simulink model "DynamicSystemFinal"  (R2021a)
settings: Solver=VariableStepAuto  StartTime=0.0  StopTime=300  RelTol=1e-3
values from neighbouring files (symbols this model uses):
  res = zeros(1, 2)    [AutonomousVehicle.m]    (also in trajectory_final_2.m)
  speed = zeros(K-1,1)    [AutonomousVehicle.m]    (also in trajectory_final_2.m)
undefined symbols (not defined in the file or in its folder): DiscIntNeverNeededParam
libraries: simulink x5, pid_lib x2, dspswit3 x1, mcbcontrolslib x1
settings Model: Creator=admin  LastModifiedBy=admin

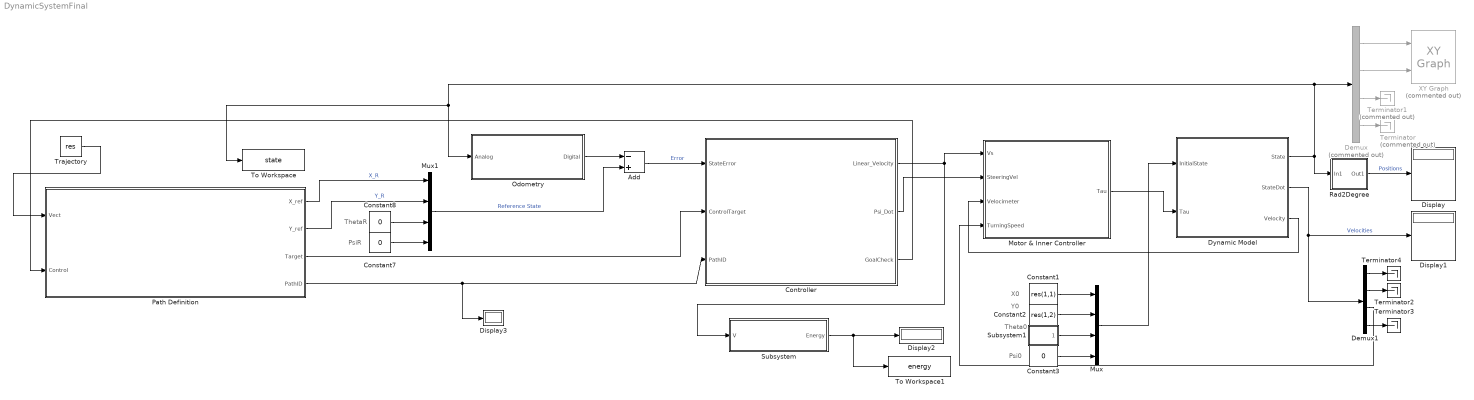
== system DynamicSystemFinal ==
  note: PsiR
  note: ThetaR
  note: Psi0
  note: Theta0
  note: X0
  note: Y0
  Add : Sum  Inputs=-+
  Constant1 : Constant  Value=res(1,1)  VectorParams1D=off  SampleTime=0.001
  Constant2 : Constant  Value=res(1,2)  SampleTime=0.001
  Constant3 : Constant  Value=0  SampleTime=0.001
  Constant7 : Constant  Value=0  SampleTime=0.001
  Constant8 : Constant  Value=0  SampleTime=0.001
  Controller : Subsystem
  Demux : Demux  Commented=on
  Demux1 : Demux
  Display{,1..3} (4 alike) : Display
  Dynamic Model : Subsystem
  Motor & Inner Controller : Subsystem
  Mux : Mux
  Mux1 : Mux
  Odometry : Subsystem
  Path Definition : Subsystem
  Rad2Degree : Subsystem
  Subsystem : Subsystem
  Subsystem1 : Subsystem
  Terminator : Terminator  Commented=on
  Terminator1 : Terminator  Commented=on
  Terminator2 : Terminator
  Terminator3 : Terminator
  Terminator4 : Terminator
  To Workspace : ToWorkspace  VariableName=state  SampleTime=0.001
      settings: Save2DSignal=2-D array (concatenate along first dimension)
  To Workspace1 : ToWorkspace  VariableName=energy  SaveFormat=Timeseries  SampleTime=0.001
      settings: MaxDataPoints=1
  Trajectory : Constant  Value=res
  XY Graph : simulink/Sinks/XY Graph  Commented=on  xmin=0  xmax=400  ymin=0  ymax=700  st=inf
  wires:
  Path Definition/4(PathID) -> Controller/3(PathID), Display3/1
  Demux/3 -> Terminator1/1
  Path Definition/3(Target) -> Controller/2(ControlTarget)
  Path Definition/1(X_ref) -> Mux1/1  "X_R"
  Add/1 -> Controller/1(StateError)  "Error"
  Controller/2(Psi_Dot) -> Motor & Inner Controller/2(SteeringVel)
  Dynamic Model/1(State) -> Rad2Degree/1(In1), Odometry/1(Analog), To Workspace/1, Demux/1
  Controller/1(Linear_Velocity) -> Motor & Inner Controller/1(Vs), Subsystem/1(V)
  Odometry/1(Digital) -> Add/1
  Constant2/1 -> Mux/2
  Rad2Degree/1(Out1) -> Display/1  "Positions"
  Mux1/1 -> Add/2  "Reference State"
  Path Definition/2(Y_ref) -> Mux1/2  "Y_R"
  Demux/4 -> Terminator/1
  Trajectory/1 -> Path Definition/1(Vect)
  Demux/1 -> XY Graph/1
  Subsystem/1(Energy) -> To Workspace1/1, Display2/1
  Demux/2 -> XY Graph/2
  Constant8/1 -> Mux1/3
  Mux/1 -> Dynamic Model/1(InitialState)
  Subsystem1/1(Theta0) -> Mux/3
  Constant7/1 -> Mux1/4
  Controller/3(GoalCheck) -> Path Definition/2(Control)
  Constant1/1 -> Mux/1
  Dynamic Model/2(StateDot) -> Demux1/1, Display1/1  "Velocities"
  Constant3/1 -> Mux/4
  Motor & Inner Controller/1(Tau) -> Dynamic Model/2(Tau)
  Dynamic Model/3(Velocity) -> Motor & Inner Controller/3(Velocimeter)
  Demux1/4 -> Terminator3/1
  Demux1/2 -> Terminator2/1
  Demux1/1 -> Terminator4/1
  Demux1/3 -> Motor & Inner Controller/4(TurningSpeed)

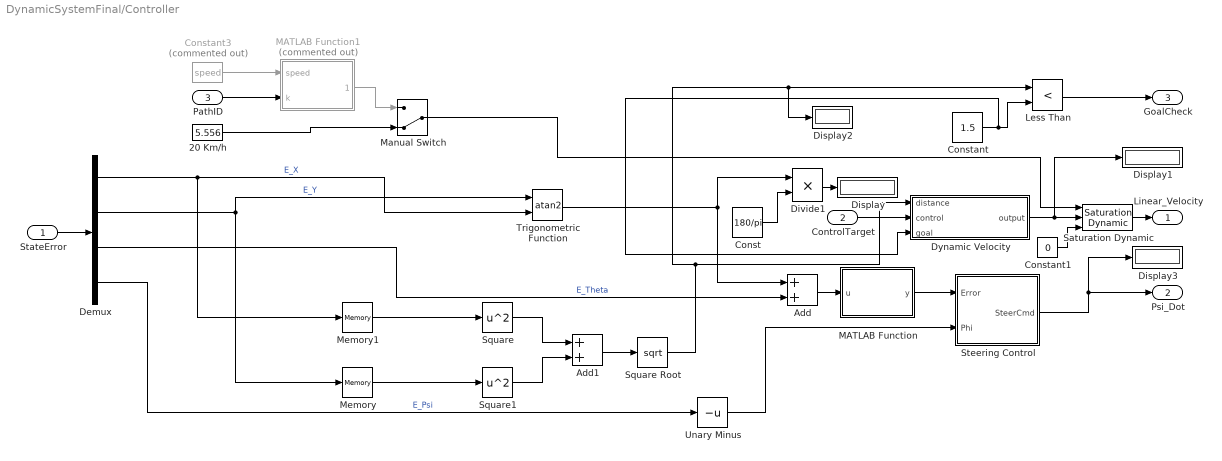
== system DynamicSystemFinal/Controller ==
  StateError : Inport
  ControlTarget : Inport  Port=2
  PathID : Inport  Port=3
  20 Km/h : Constant  Value=5.556
  Add : Sum
  Add1 : Sum
  Const : Constant  Value=180/pi
  Constant : Constant  Value=1.5  SampleTime=0.001
  Constant1 : Constant  Value=0
  Constant3 : Constant  Commented=on  Value=speed
  Demux : Demux
  Display{,1..3} (4 alike) : Display
  Divide1 : Product  Inputs=**
  Dynamic Velocity : Subsystem
  Less Than : RelationalOperator  Operator=<  OutDataTypeStr=boolean  RndMeth=Simplest
  MATLAB Function : MATLAB Function  TreatAsAtomicUnit=on
  MATLAB Function1 : MATLAB Function  Commented=on  TreatAsAtomicUnit=on
  Manual Switch : ManualSwitch  CurrentSetting=0
  Memory : Memory
  Memory1 : Memory
  Saturation Dynamic : simulink/Discontinuities/Saturation Dynamic  OutMin=[]  OutMax=[]  OutDataTypeStr=Inherit: Same as second input  OutDataType=fixdt(1, 16)  OutScaling=2^-10  DoSatur=off
  Square : Math  Operator=square  SaturateOnIntegerOverflow=on
  Square Root : Sqrt  SaturateOnIntegerOverflow=on
  Square1 : Math  Operator=square  SaturateOnIntegerOverflow=on
  Steering Control : Subsystem
  Trigonometric Function : Trigonometry  Operator=atan2
  Unary Minus : UnaryMinus
  Linear_Velocity : Outport
  Psi_Dot : Outport  Port=2
  GoalCheck : Outport  Port=3
  wires:
  StateError/1 -> Demux/1
  Demux/2 -> Trigonometric Function/1, Memory/1  "E_Y"
  Demux/3 -> Add/2  "E_Theta"
  Demux/1 -> Trigonometric Function/2, Memory1/1  "E_X"
  Constant/1 -> Dynamic Velocity/3(goal), Less Than/2
  Less Than/1 -> GoalCheck/1
  Square/1 -> Add1/1
  Square1/1 -> Add1/2
  Add1/1 -> Square Root/1
  Add/1 -> MATLAB Function/1(u)
  Const/1 -> Divide1/2
  Divide1/1 -> Display/1
  Square Root/1 -> Dynamic Velocity/1(distance), Less Than/1, Display2/1
  Dynamic Velocity/1(output) -> Display1/1, Saturation Dynamic/2
  ControlTarget/1 -> Dynamic Velocity/2(control)
  Memory/1 -> Square1/1
  Memory1/1 -> Square/1
  Saturation Dynamic/1 -> Linear_Velocity/1
  Constant1/1 -> Saturation Dynamic/3
  Manual Switch/1 -> Saturation Dynamic/1
  20 Km/h/1 -> Manual Switch/2
  Constant3/1 -> MATLAB Function1/1(speed)
  PathID/1 -> MATLAB Function1/2(k)
  MATLAB Function1/1(max_vel) -> Manual Switch/1
  Trigonometric Function/1 -> Divide1/1, Add/1
  Demux/4 -> Unary Minus/1  "E_Psi"
  Steering Control/1(SteerCmd) -> Display3/1, Psi_Dot/1
  MATLAB Function/1(y) -> Steering Control/1(Error)
  Unary Minus/1 -> Steering Control/2(Phi)

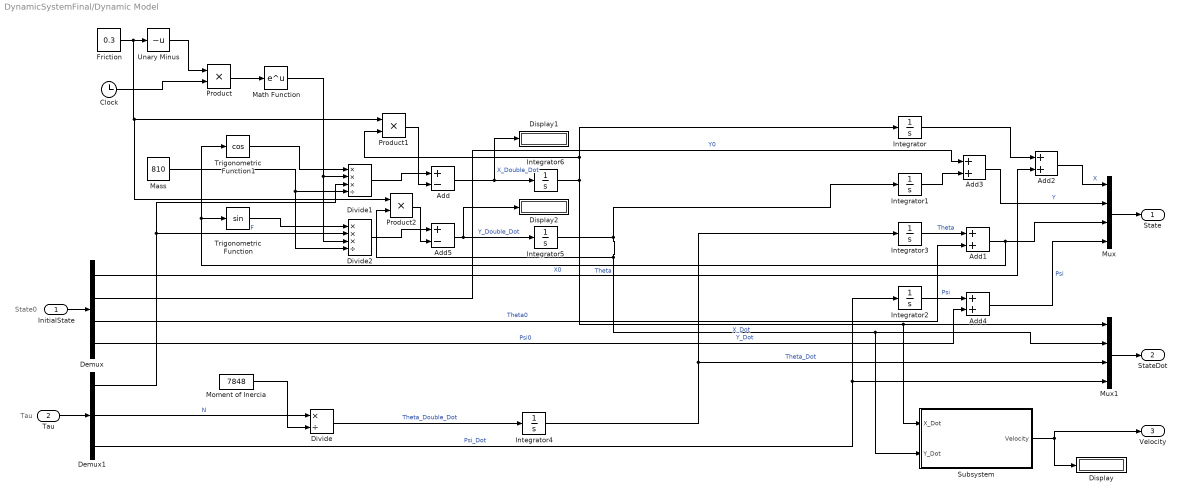
== system DynamicSystemFinal/Dynamic Model ==
  note: Tau
  note: State0
  InitialState : Inport
  Tau : Inport  Port=2
  Add : Sum  Inputs=+-
  Add{1..4} (4 alike) : Sum
  Add5 : Sum  Inputs=+-
  Clock : Clock
  Demux : Demux
  Demux1 : Demux  Outputs=3
  Display : Display
  Display1 : Display
  Display2 : Display
  Divide : Product  Inputs=*/
  Divide1 : Product  Inputs=***/
  Divide2 : Product  Inputs=***/
  Friction : Constant  Value=0.3
  Integrator{,1..6} (7 alike) : Integrator
  Mass : Constant  Value=810
  Math Function : Math  SaturateOnIntegerOverflow=on
  Moment of Inercia : Constant  Value=7848
  Mux : Mux
  Mux1 : Mux
  Product : Product
  Product1 : Product
  Product2 : Product
  Subsystem : Subsystem
  Trigonometric Function : Trigonometry
  Trigonometric Function1 : Trigonometry  Operator=cos
  Unary Minus : UnaryMinus
  State : Outport
  StateDot : Outport  Port=2
  Velocity : Outport  Port=3
  wires:
  Mux/1 -> State/1
  Mux1/1 -> StateDot/1
  Demux1/3 -> Integrator2/1, Mux1/4  "Psi_Dot"
  Add4/1 -> Mux/4  "Psi"
  Add1/1 -> Trigonometric Function/1, Trigonometric Function1/1, Mux/3  "Theta"
  Integrator/1 -> Add2/1
  InitialState/1 -> Demux/1
  Add2/1 -> Mux/1  "X"
  Integrator1/1 -> Add3/2
  Add3/1 -> Mux/2  "Y"
  Tau/1 -> Demux1/1
  Demux/2 -> Add3/1  "Y0"
  Demux/1 -> Add2/2  "X0"
  Integrator3/1 -> Add1/1  "Theta"
  Demux/3 -> Add1/2  "Theta0"
  Integrator2/1 -> Add4/1  "Psi"
  Demux/4 -> Add4/2  "Psi0"
  Moment of Inercia/1 -> Divide/2
  Divide/1 -> Integrator4/1  "Theta_Double_Dot"
  Integrator4/1 -> Integrator3/1, Mux1/3  "Theta_Dot"
  Add/1 -> Display1/1, Integrator6/1  "X_Double_Dot"
  Add5/1 -> Display2/1, Integrator5/1  "Y_Double_Dot"
  Demux1/2 -> Divide/1  "N"
  Trigonometric Function1/1 -> Divide1/1
  Trigonometric Function/1 -> Divide2/1
  Mass/1 -> Divide1/4, Divide2/4
  Demux1/1 -> Divide1/3, Divide2/2  "F"
  Integrator5/1 -> Product2/2, Subsystem/2(Y_Dot), Mux1/2, Integrator1/1  "Y_Dot"
  Integrator6/1 -> Product1/2, Integrator/1, Mux1/1, Subsystem/1(X_Dot)  "X_Dot"
  Subsystem/1(Velocity) -> Display/1, Velocity/1
  Clock/1 -> Product/2
  Friction/1 -> Product2/1, Product1/1, Unary Minus/1
  Unary Minus/1 -> Product/1
  Product/1 -> Math Function/1
  Math Function/1 -> Divide2/3, Divide1/2
  Divide1/1 -> Add/1
  Product1/1 -> Add/2
  Divide2/1 -> Add5/1
  Product2/1 -> Add5/2

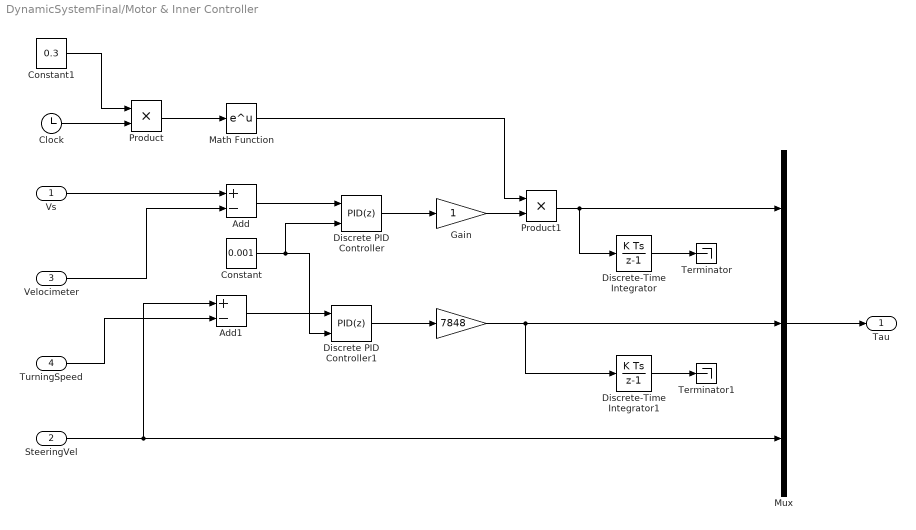
== system DynamicSystemFinal/Motor & Inner Controller ==
  Vs : Inport
  SteeringVel : Inport  Port=2
  Velocimeter : Inport  Port=3
  TurningSpeed : Inport  Port=4
  " " : Gain  Gain=7848
  Add : Sum  Inputs=+-
  Add1 : Sum  Inputs=+-
  Clock : Clock
  Constant : Constant  Value=0.001
  Constant1 : Constant  Value=0.3
  Discrete PID Controller : pid_lib/PID Controller  Controller=PID  Form=Parallel  TimeDomain=Discrete-time  UseExternalTs=on  SampleTime=-1  IntegratorMethod=Forward Euler  FilterMethod=Forward Euler  ControllerParametersSource=internal  P=1  I=30  D=0  UseFilter=on  N=100  TunerSelectOption=Transfer Function Based (PID Tuner App)  InitialConditionSource=internal  InitialConditionForIntegrator=0  InitialConditionForFilter=0  DifferentiatorICPrevScaledInput=0  ExternalReset=none  TrackingMode=off  Kt=1  LimitOutput=off  SatLimitsSource=internal  UpperSaturationLimit=inf  LowerSaturationLimit=-inf  LinearizeAsGain=off  AntiWindupMode=none  Kb=1  POutMin=[]  POutMax=[]  IOutMin=[]  IOutMax=[]  DOutMin=[]  DOutMax=[]  NOutMin=[]  NOutMax=[]  SumOutMin=[]  SumOutMax=[]  SaturationOutMin=[]  SaturationOutMax=[]  PParamMin=[]  PParamMax=[]  IParamMin=[]  IParamMax=[]  DParamMin=[]  DParamMax=[]  NParamMin=[]  NParamMax=[]  KbParamMin=[]  KbParamMax=[]  KtParamMin=[]  KtParamMax=[]  KbOutMin=[]  KbOutMax=[]  KtOutMin=[]  KtOutMax=[]  IntegratorOutMin=[]  IntegratorOutMax=[]  FilterOutMin=[]  FilterOutMax=[]  SumI1OutMin=[]  SumI1OutMax=[]  SumI2OutMin=[]  SumI2OutMax=[]  SumI3OutMin=[]  SumI3OutMax=[]  SumI4OutMin=[]  SumI4OutMax=[]  SumDOutMin=[]  SumDOutMax=[]  DifferentiatorOutMin=[]  DifferentiatorOutMax=[]  FilterDiffOutCoefMin=[]  FilterDiffOutCoefMax=[]  ReciprocalOutMin=[]  ReciprocalOutMax=[]  SumDenOutMin=[]  SumDenOutMax=[]  SumNumOutMin=[]  SumNumOutMax=[]  DivideOutMin=[]  DivideOutMax=[]  UdiffTsProdOutMin=[]  UdiffTsProdOutMax=[]  NTsProdOutMin=[]  NTsProdOutMax=[]  UintegralTsProdOutMin=[]  UintegralTsProdOutMax=[]  UngainTsProdOutMin=[]  UngainTsProdOutMax=[]  IntegratorContinuousStateAttributes=''  IntegratorStateMustResolveToSignalObject=off  IntegratorRTWStateStorageClass=Auto  FilterContinuousStateAttributes=''  FilterStateMustResolveToSignalObject=off  FilterRTWStateStorageClass=Auto  ParallelPVariant=InternalParameters  IdealPVariant=Disabled  IVariant=InternalParameters  DVariant=InternalParameters  IntegratorVariant=Discrete  SatVariant=Disabled  AWVariant=Passthrough  PCopyVariant=Disabled  TRVariant=Disabled  FdbkBlocksVariant=Forward  IdealPFdbkVariant=Disabled  SatFdbkVariant=Disabled  DerivativeFilterVariant=ForwardEulerFilter  NVariant=InternalParameters  NCopyVariant=Disabled  FilterICVariant=InternalICsFilter  IntegratorICVariant=InternalICs  ExternalResetVariant=Disabled  TRSumVariant=Passthrough  SumFdbkVariant=Disabled  SumVariant=Sum_PID  TsampFilterVariant=ExternalTs  TsampNgainVariant=ExternalTs  TsampIntegralVariant=ExternalTs  ExternalSaturationOutDataTypeStr=Inherit: Same as second input
  Discrete PID Controller1 : pid_lib/PID Controller  Controller=PID  Form=Parallel  TimeDomain=Discrete-time  UseExternalTs=on  SampleTime=-1  IntegratorMethod=Forward Euler  FilterMethod=Forward Euler  ControllerParametersSource=internal  P=1  I=1  D=0  UseFilter=on  N=100  TunerSelectOption=Transfer Function Based (PID Tuner App)  InitialConditionSource=internal  InitialConditionForIntegrator=0  InitialConditionForFilter=0  DifferentiatorICPrevScaledInput=0  ExternalReset=none  TrackingMode=off  Kt=1  LimitOutput=off  SatLimitsSource=internal  UpperSaturationLimit=inf  LowerSaturationLimit=-inf  LinearizeAsGain=off  AntiWindupMode=none  Kb=1  POutMin=[]  POutMax=[]  IOutMin=[]  IOutMax=[]  DOutMin=[]  DOutMax=[]  NOutMin=[]  NOutMax=[]  SumOutMin=[]  SumOutMax=[]  SaturationOutMin=[]  SaturationOutMax=[]  PParamMin=[]  PParamMax=[]  IParamMin=[]  IParamMax=[]  DParamMin=[]  DParamMax=[]  NParamMin=[]  NParamMax=[]  KbParamMin=[]  KbParamMax=[]  KtParamMin=[]  KtParamMax=[]  KbOutMin=[]  KbOutMax=[]  KtOutMin=[]  KtOutMax=[]  IntegratorOutMin=[]  IntegratorOutMax=[]  FilterOutMin=[]  FilterOutMax=[]  SumI1OutMin=[]  SumI1OutMax=[]  SumI2OutMin=[]  SumI2OutMax=[]  SumI3OutMin=[]  SumI3OutMax=[]  SumI4OutMin=[]  SumI4OutMax=[]  SumDOutMin=[]  SumDOutMax=[]  DifferentiatorOutMin=[]  DifferentiatorOutMax=[]  FilterDiffOutCoefMin=[]  FilterDiffOutCoefMax=[]  ReciprocalOutMin=[]  ReciprocalOutMax=[]  SumDenOutMin=[]  SumDenOutMax=[]  SumNumOutMin=[]  SumNumOutMax=[]  DivideOutMin=[]  DivideOutMax=[]  UdiffTsProdOutMin=[]  UdiffTsProdOutMax=[]  NTsProdOutMin=[]  NTsProdOutMax=[]  UintegralTsProdOutMin=[]  UintegralTsProdOutMax=[]  UngainTsProdOutMin=[]  UngainTsProdOutMax=[]  IntegratorContinuousStateAttributes=''  IntegratorStateMustResolveToSignalObject=off  IntegratorRTWStateStorageClass=Auto  FilterContinuousStateAttributes=''  FilterStateMustResolveToSignalObject=off  FilterRTWStateStorageClass=Auto  ParallelPVariant=InternalParameters  IdealPVariant=Disabled  IVariant=InternalParameters  DVariant=InternalParameters  IntegratorVariant=Discrete  SatVariant=Disabled  AWVariant=Passthrough  PCopyVariant=Disabled  TRVariant=Disabled  FdbkBlocksVariant=Forward  IdealPFdbkVariant=Disabled  SatFdbkVariant=Disabled  DerivativeFilterVariant=ForwardEulerFilter  NVariant=InternalParameters  NCopyVariant=Disabled  FilterICVariant=InternalICsFilter  IntegratorICVariant=InternalICs  ExternalResetVariant=Disabled  TRSumVariant=Passthrough  SumFdbkVariant=Disabled  SumVariant=Sum_PID  TsampFilterVariant=ExternalTs  TsampNgainVariant=ExternalTs  TsampIntegralVariant=ExternalTs  ExternalSaturationOutDataTypeStr=Inherit: Same as second input
  Discrete-Time Integrator : DiscreteIntegrator  gainval=1/810  SampleTime=-1  ICPrevOutput=DiscIntNeverNeededParam  ICPrevScaledInput=DiscIntNeverNeededParam
  Discrete-Time Integrator1 : DiscreteIntegrator  gainval=1/7848  SampleTime=-1  ICPrevOutput=DiscIntNeverNeededParam  ICPrevScaledInput=DiscIntNeverNeededParam
  Gain : Gain
  Math Function : Math  SaturateOnIntegerOverflow=on
  Mux : Mux  Inputs=3
  Product : Product
  Product1 : Product
  Terminator : Terminator
  Terminator1 : Terminator
  Tau : Outport
  wires:
  Mux/1 -> Tau/1
  SteeringVel/1 -> Add1/1, Mux/3
  Discrete PID Controller/1 -> Gain/1
  Product1/1 -> Mux/1, Discrete-Time Integrator/1
  Add1/1 -> Discrete PID Controller1/1
  Add/1 -> Discrete PID Controller/1
  Vs/1 -> Add/1
  Discrete-Time Integrator/1 -> Terminator/1
  Constant/1 -> Discrete PID Controller/2, Discrete PID Controller1/2
  Discrete PID Controller1/1 -> " "/1
  " "/1 -> Discrete-Time Integrator1/1, Mux/2
  Velocimeter/1 -> Add/2
  Constant1/1 -> Product/1
  Clock/1 -> Product/2
  Product/1 -> Math Function/1
  Gain/1 -> Product1/2
  Math Function/1 -> Product1/1
  Discrete-Time Integrator1/1 -> Terminator1/1
  TurningSpeed/1 -> Add1/2

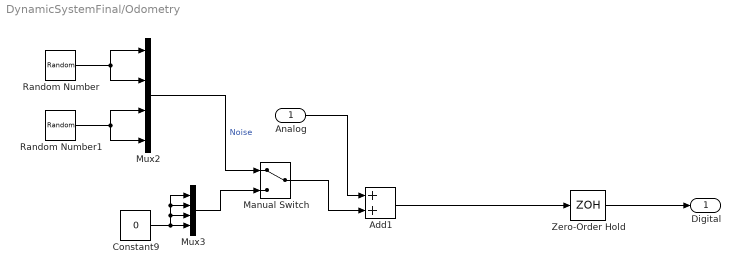
== system DynamicSystemFinal/Odometry ==
  Analog : Inport
  Add1 : Sum
  Constant9 : Constant  Value=0  SampleTime=0.001
  Manual Switch : ManualSwitch
  Mux2 : Mux
  Mux3 : Mux
  Random Number : RandomNumber  Variance=0.005  SampleTime=0.001
  Random Number1 : RandomNumber  Variance=0.002  SampleTime=0.001
  Zero-Order Hold : ZeroOrderHold  SampleTime=-1
  Digital : Outport
  wires:
  Constant9/1 -> Mux3/2, Mux3/1, Mux3/3, Mux3/4
  Random Number1/1 -> Mux2/4, Mux2/3
  Random Number/1 -> Mux2/1, Mux2/2
  Mux3/1 -> Manual Switch/2
  Mux2/1 -> Manual Switch/1  "Noise"
  Add1/1 -> Zero-Order Hold/1
  Manual Switch/1 -> Add1/2
  Analog/1 -> Add1/1
  Zero-Order Hold/1 -> Digital/1

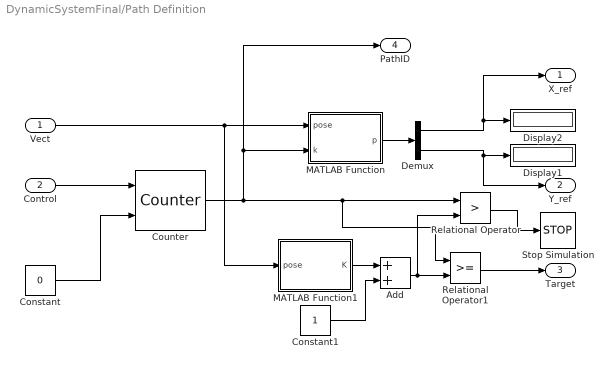
== system DynamicSystemFinal/Path Definition ==
  Vect : Inport
  Control : Inport  Port=2
  Add : Sum
  Constant : Constant  Value=0
  Constant1 : Constant
  Counter : dspswit3/Counter  Direction=Up  CountEvent=Rising edge  CounterSize=User defined  MaxCount=255  InitialCount=2  Output=Count  HitValue=32  ResetInput=on  SamplesPerFrame=1  Ts=1  CntDtype=double  HitDtype=Logical
  Demux : Demux  Outputs=2
  Display1 : Display
  Display2 : Display
  MATLAB Function : MATLAB Function  TreatAsAtomicUnit=on
  MATLAB Function1 : MATLAB Function  TreatAsAtomicUnit=on
  Relational Operator : RelationalOperator  Operator=>  OutDataTypeStr=boolean  RndMeth=Simplest
  Relational Operator1 : RelationalOperator  OutDataTypeStr=boolean  RndMeth=Simplest
  Stop Simulation : Stop
  X_ref : Outport
  Y_ref : Outport  Port=2
  Target : Outport  Port=3
  PathID : Outport  Port=4
  wires:
  Vect/1 -> MATLAB Function1/1(pose), MATLAB Function/1(pose)
  MATLAB Function/1(p) -> Demux/1
  Demux/1 -> X_ref/1, Display2/1
  Demux/2 -> Y_ref/1, Display1/1
  Constant/1 -> Counter/2
  Control/1 -> Counter/1
  Add/1 -> Relational Operator1/2, Relational Operator/2
  Relational Operator1/1 -> Target/1
  Relational Operator/1 -> Stop Simulation/1
  Counter/1 -> Relational Operator1/1, Relational Operator/1, PathID/1, MATLAB Function/2(k)
  Constant1/1 -> Add/2
  MATLAB Function1/1(K) -> Add/1

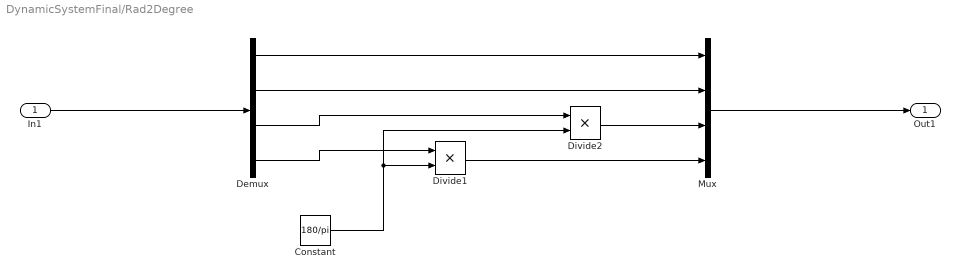
== system DynamicSystemFinal/Rad2Degree ==
  In1 : Inport
  Constant : Constant  Value=180/pi
  Demux : Demux
  Divide1 : Product  Inputs=**
  Divide2 : Product  Inputs=**
  Mux : Mux
  Out1 : Outport
  wires:
  In1/1 -> Demux/1
  Mux/1 -> Out1/1
  Demux/1 -> Mux/1
  Demux/2 -> Mux/2
  Demux/3 -> Divide2/1
  Demux/4 -> Divide1/1
  Constant/1 -> Divide1/2, Divide2/2
  Divide1/1 -> Mux/4
  Divide2/1 -> Mux/3

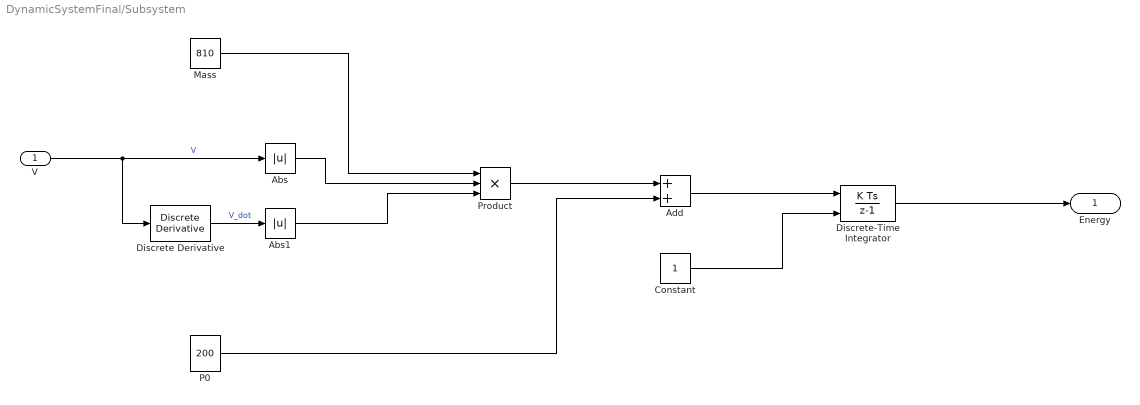
== system DynamicSystemFinal/Subsystem ==
  V : Inport
  Abs : Abs
  Abs1 : Abs
  Add : Sum
  Constant : Constant
  Discrete Derivative : simulink/Discrete/Discrete Derivative  gainval=1.0  ICPrevScaledInput=1  OutMin=[]  OutMax=[]  OutDataType=fixdt(1, 16)  OutScaling=2^-10  DoSatur=off
  Discrete-Time Integrator : DiscreteIntegrator  InitialConditionSource=external  SampleTime=0.01  ICPrevOutput=DiscIntNeverNeededParam  ICPrevScaledInput=DiscIntNeverNeededParam
  Mass : Constant  Value=810
  P0 : Constant  Value=200
  Product : Product  Inputs=3
  Energy : Outport
  wires:
  Discrete-Time Integrator/1 -> Energy/1
  Product/1 -> Add/1
  P0/1 -> Add/2
  Add/1 -> Discrete-Time Integrator/1
  V/1 -> Abs/1, Discrete Derivative/1  "V"
  Mass/1 -> Product/1
  Constant/1 -> Discrete-Time Integrator/2
  Discrete Derivative/1 -> Abs1/1  "V_dot"
  Abs/1 -> Product/2
  Abs1/1 -> Product/3

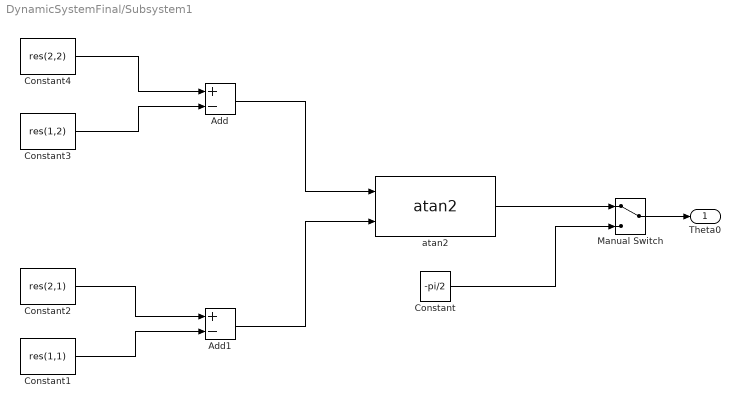
== system DynamicSystemFinal/Subsystem1 ==
  Add : Sum  Inputs=+-
  Add1 : Sum  Inputs=+-
  Constant : Constant  Value=-pi/2
  Constant1 : Constant  Value=res(1,1)
  Constant2 : Constant  Value=res(2,1)
  Constant3 : Constant  Value=res(1,2)
  Constant4 : Constant  Value=res(2,2)
  Manual Switch : ManualSwitch
  atan2 : mcbcontrolslib/atan2  outputUnit=Radians
      settings: SourceProductBaseCode=MT
  Theta0 : Outport
  wires:
  atan2/1 -> Manual Switch/1
  Constant3/1 -> Add/2
  Constant4/1 -> Add/1
  Constant2/1 -> Add1/1
  Constant1/1 -> Add1/2
  Add1/1 -> atan2/2
  Add/1 -> atan2/1
  Manual Switch/1 -> Theta0/1
  Constant/1 -> Manual Switch/2

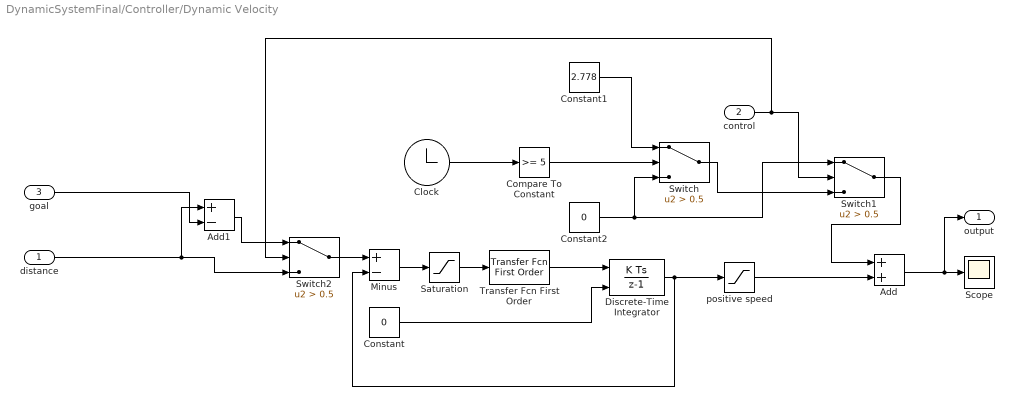
== system DynamicSystemFinal/Controller/Dynamic Velocity ==
  distance : Inport
  control : Inport  Port=2
  goal : Inport  Port=3
  Add : Sum
  Add1 : Sum  Inputs=+-
  Clock : Clock
  Compare To Constant : simulink/Logic and Bit Operations/Compare To Constant  relop=>=  const=5  OutDataTypeStr=boolean
  Constant : Constant  Value=0
  Constant1 : Constant  Value=2.778
  Constant2 : Constant  Value=0
  Discrete-Time Integrator : DiscreteIntegrator  gainval=6  InitialConditionSource=external  SampleTime=0.001  ICPrevOutput=DiscIntNeverNeededParam  ICPrevScaledInput=DiscIntNeverNeededParam
  Minus : Sum  Inputs=+-
  Saturation : Saturate  UpperLimit=2  LowerLimit=-10
  Scope : Scope
  Switch : Switch  Criteria=u2 > Threshold  Threshold=0.5
  Switch1 : Switch  Criteria=u2 > Threshold  Threshold=0.5
  Switch2 : Switch  Criteria=u2 > Threshold  Threshold=0.5
  Transfer Fcn First Order : simulink/Discrete/Transfer Fcn First Order  PoleZ=0.998  ICPrevOutput=0.0  DoSatur=off
  positive speed : Saturate  UpperLimit=inf  LowerLimit=0
  output : Outport
  wires:
  distance/1 -> Switch2/3, Add1/1
  Add/1 -> Scope/1, output/1
  Saturation/1 -> Transfer Fcn First Order/1
  Transfer Fcn First Order/1 -> Discrete-Time Integrator/1
  Minus/1 -> Saturation/1
  Constant/1 -> Discrete-Time Integrator/2
  Discrete-Time Integrator/1 -> positive speed/1, Minus/2
  Constant2/1 -> Switch1/1, Switch/3
  Constant1/1 -> Switch/1
  Switch1/1 -> Add/1
  Compare To Constant/1 -> Switch/2
  Clock/1 -> Compare To Constant/1
  control/1 -> Switch2/2, Switch1/2
  Switch/1 -> Switch1/3
  Switch2/1 -> Minus/1
  goal/1 -> Add1/2
  Add1/1 -> Switch2/1
  positive speed/1 -> Add/2

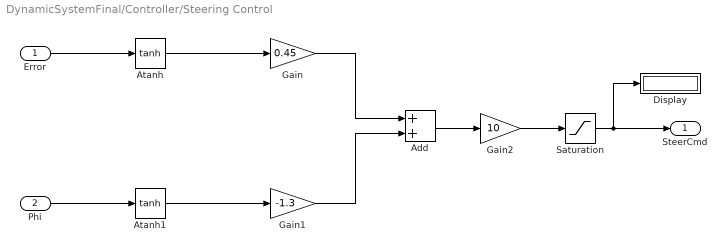
== system DynamicSystemFinal/Controller/Steering Control ==
  Error : Inport
  Phi : Inport  Port=2
  Add : Sum
  Atanh : Trigonometry  Operator=tanh
  Atanh1 : Trigonometry  Operator=tanh
  Display : Display
  Gain : Gain  Gain=0.45
  Gain1 : Gain  Gain=-1.3
  Gain2 : Gain  Gain=10
  Saturation : Saturate  UpperLimit=pi/3  LowerLimit=-pi/3
  SteerCmd : Outport
  wires:
  Error/1 -> Atanh/1
  Atanh/1 -> Gain/1
  Phi/1 -> Atanh1/1
  Add/1 -> Gain2/1
  Gain/1 -> Add/1
  Atanh1/1 -> Gain1/1
  Gain1/1 -> Add/2
  Saturation/1 -> Display/1, SteerCmd/1
  Gain2/1 -> Saturation/1

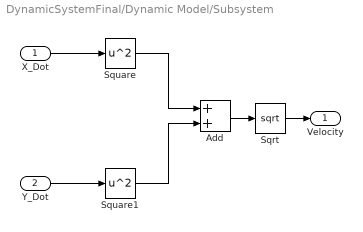
== system DynamicSystemFinal/Dynamic Model/Subsystem ==
  X_Dot : Inport
  Y_Dot : Inport  Port=2
  Add : Sum
  Sqrt : Sqrt  SaturateOnIntegerOverflow=on
  Square : Math  Operator=square  SaturateOnIntegerOverflow=on
  Square1 : Math  Operator=square  SaturateOnIntegerOverflow=on
  Velocity : Outport
  wires:
  Y_Dot/1 -> Square1/1
  X_Dot/1 -> Square/1
  Sqrt/1 -> Velocity/1
  Add/1 -> Sqrt/1
  Square/1 -> Add/1
  Square1/1 -> Add/2

== matlab function DynamicSystemFinal/Path Definition/MATLAB Function ==
  data: pose input; p output; k input
function p = fcn(pose, k)

[S,~] = size(pose);

if k>(S+1)
    u = S; 
elseif k<=0
    u = 1;
else
    u = k;
end

p = pose(uint8(u),:);

== matlab function DynamicSystemFinal/Path Definition/MATLAB Function1 ==
  data: pose input; K output
function K = fcn(pose)
[S,~] = size(pose);
K = S;

== matlab function DynamicSystemFinal/Controller/MATLAB Function1 ==
  data: speed input; max_vel output; k input
function max_vel = fcn(speed, k)
    
    [S,~] = size(speed);
    
    if k > S
        u = speed(S);
    elseif k <= 0
        u = speed(1);
    else
        u = speed(k);
    end

max_vel = u;

== matlab function DynamicSystemFinal/Controller/MATLAB Function ==
  data: u input; y output
function y = fcn(u)
if u>0
    if u > pi
        K = u-2*pi;
    else
        K = u;
    end
else
    if u < -pi
        K = 2*pi+u;
    else
        K = u;
    end
end
y = K;
